simulink model "boat_sim_ss_bruce"  (R2018b)
settings: Solver=VariableStepAuto  StartTime=0.0  StopTime=20  RelTol=1e-3
undefined symbols (not defined in the file or in its folder): linearized_B_disturb, state_eq
(part 1 of 2)
settings Model: Creator=brucecui  LastModifiedBy=bruce

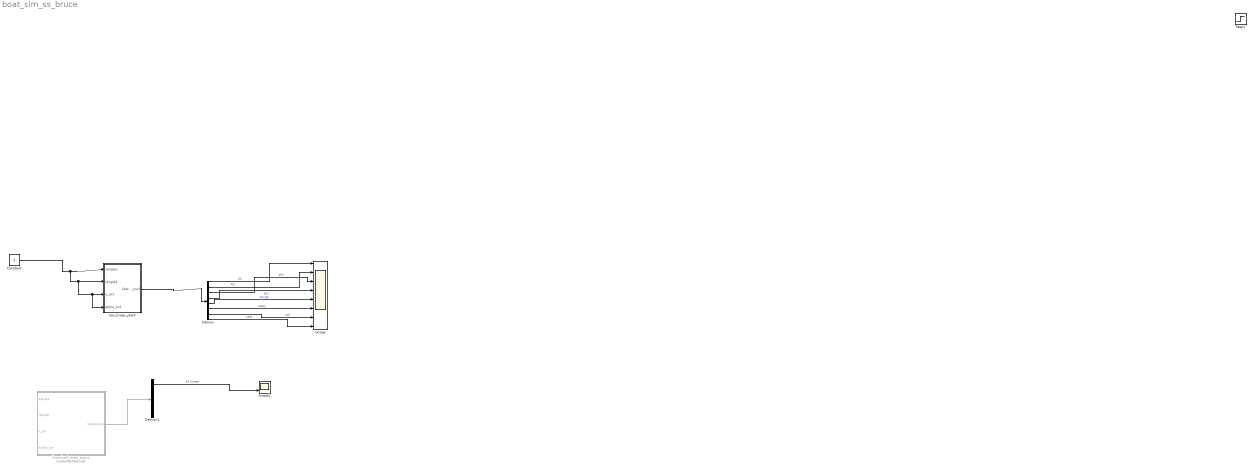
== system boat_sim_ss_bruce ==
  Constant : Constant
  Demux : Demux  Outputs=8
  Demux1 : Demux  Outputs=8
  Scope : Scope  NumInputPorts=8
  Scope1 : Scope  NumInputPorts=2
  Step1 : Step  Time=0  SampleTime=0
  linearized_state_space : Subsystem  Commented=on
  non_linear_plant : Subsystem
  wires:
  non_linear_plant/1(States_out1) -> Demux/1
  linearized_state_space/1(States_out) -> Demux1/1
  Demux1/2 -> Scope1/2  "X2 linear"
  Demux/1 -> Scope/1  "X1"
  Demux/2 -> Scope/2  "X2"
  Demux/3 -> Scope/3  "phi"
  Demux/4 -> Scope/4  "psi"
  Demux/5 -> Scope/5  "surge"
  Demux/6 -> Scope/6  "sway"
  Demux/7 -> Scope/7  "roll"
  Demux/8 -> Scope/8  "yaw"
  Constant/1 -> non_linear_plant/4(alpha_tw1), non_linear_plant/3(v_tw1), non_linear_plant/2(rangle1), non_linear_plant/1(sangle1)

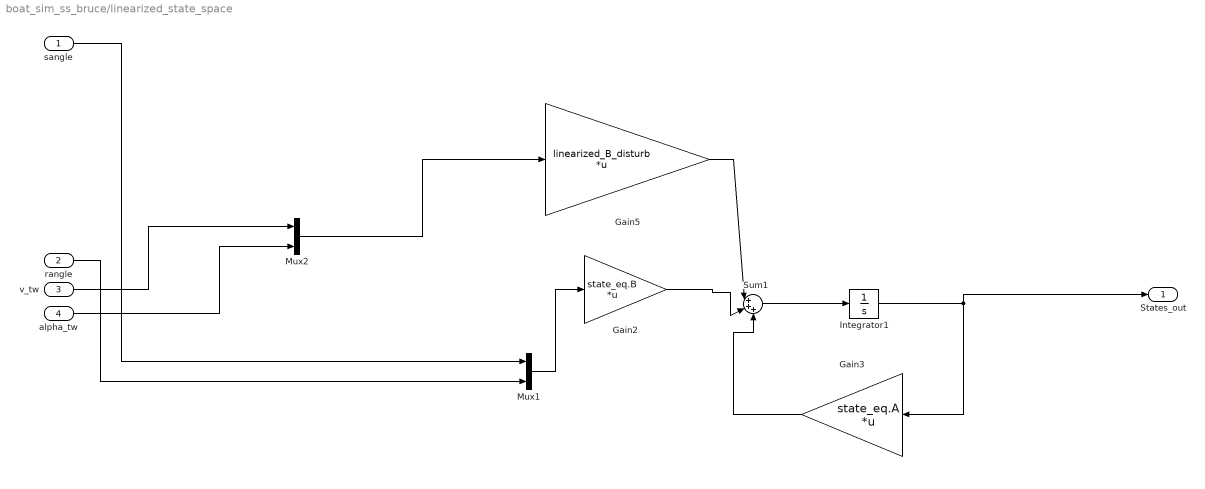
== system boat_sim_ss_bruce/linearized_state_space ==
  sangle : Inport
  rangle : Inport  Port=2
  v_tw : Inport  Port=3
  alpha_tw : Inport  Port=4
  Gain2 : Gain  Gain=state_eq.B  Multiplication=Matrix(K*u)
  Gain3 : Gain  Gain=state_eq.A  Multiplication=Matrix(K*u)
  Gain5 : Gain  Gain=linearized_B_disturb  Multiplication=Matrix(K*u)
  Integrator1 : Integrator  InitialCondition=[0 0 0 0 0 1 0 0]
  Mux1 : Mux  Inputs=2
  Mux2 : Mux  Inputs=2
  Sum1 : Sum  Inputs=|+++
  States_out : Outport
  wires:
  Integrator1/1 -> States_out/1, Gain3/1
  Gain5/1 -> Sum1/1
  Mux2/1 -> Gain5/1
  rangle/1 -> Mux1/2
  alpha_tw/1 -> Mux2/2
  sangle/1 -> Mux1/1
  v_tw/1 -> Mux2/1
  Sum1/1 -> Integrator1/1
  Mux1/1 -> Gain2/1
  Gain2/1 -> Sum1/2
  Gain3/1 -> Sum1/3

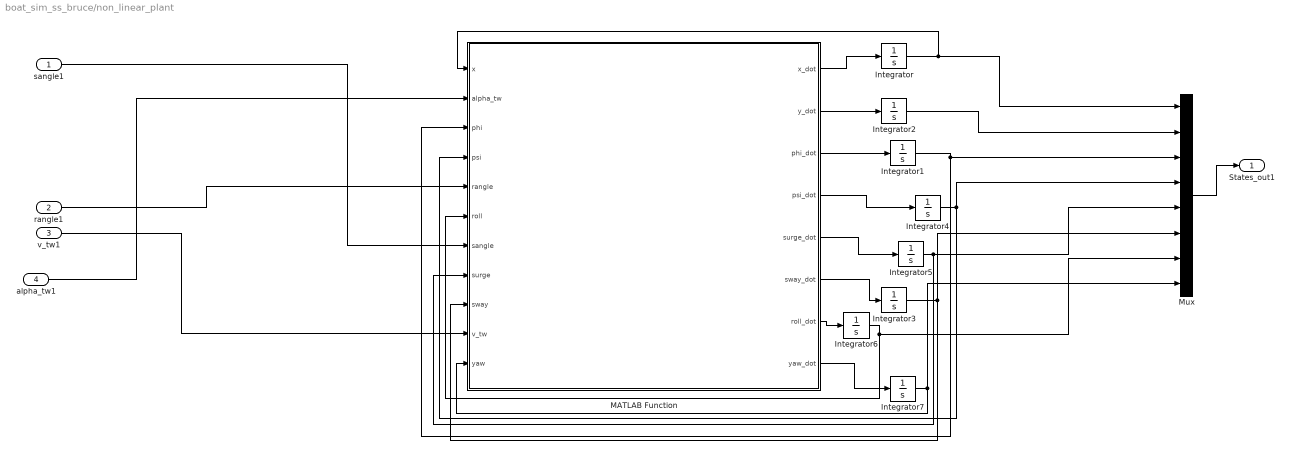
== system boat_sim_ss_bruce/non_linear_plant ==
  sangle1 : Inport
  rangle1 : Inport  Port=2
  v_tw1 : Inport  Port=3
  alpha_tw1 : Inport  Port=4
  Integrator{,1..2,4..7} (7 alike) : Integrator
  Integrator3 : Integrator  InitialCondition=10^(-60)
  MATLAB Function : MATLAB Function  TreatAsAtomicUnit=on
  Mux : Mux  Inputs=8
  States_out1 : Outport
  wires:
  alpha_tw1/1 -> MATLAB Function/2(alpha_tw)
  Integrator6/1 -> Mux/7, MATLAB Function/6(roll)
  v_tw1/1 -> MATLAB Function/10(v_tw)
  Integrator3/1 -> Mux/6, MATLAB Function/9(sway)
  Integrator/1 -> MATLAB Function/1(x), Mux/1
  Integrator1/1 -> MATLAB Function/3(phi), Mux/3
  Mux/1 -> States_out1/1
  MATLAB Function/6(sway_dot) -> Integrator3/1
  Integrator7/1 -> MATLAB Function/11(yaw), Mux/8
  Integrator4/1 -> MATLAB Function/4(psi), Mux/4
  MATLAB Function/2(y_dot) -> Integrator2/1
  MATLAB Function/1(x_dot) -> Integrator/1
  MATLAB Function/3(phi_dot) -> Integrator1/1
  MATLAB Function/7(roll_dot) -> Integrator6/1
  MATLAB Function/5(surge_dot) -> Integrator5/1
  MATLAB Function/8(yaw_dot) -> Integrator7/1
  Integrator5/1 -> Mux/5, MATLAB Function/8(surge)
  MATLAB Function/4(psi_dot) -> Integrator4/1
  rangle1/1 -> MATLAB Function/5(rangle)
  sangle1/1 -> MATLAB Function/7(sangle)
  Integrator2/1 -> Mux/2
